simulink model "sim_A3_nonlinear"  (R2022b)
settings: Solver=ode45  StartTime=0.0  StopTime=Tf  RelTol=1e-3
values from neighbouring files (symbols this model uses):
  B = diag([1 2])    [main_A3_nonlinear.m]
  controller = 4    [main_A3_nonlinear.m]
  Cs = [0.4, 0.001 ... (first row only)    [main_A3_nonlinear.m]
  gamma = 1    [main_A3_nonlinear.m]
  K1 = place(A,B,poles_cont)    [main_A3_nonlinear.m]
  K2 = [alpha 0 ... (first row only)    [main_A3_nonlinear.m]
  Ts = 1/1000    (= 0.001)    [main_A3_nonlinear.m]
  x1_o = ro * cos(k * pi/6)    [main_A3_nonlinear.m]
  x2_o = ro * sin(k * pi/6)    [main_A3_nonlinear.m]
undefined symbols (not defined in the file or in its folder): K3
settings Model: Creator=ricardoaguilera  LastModifiedBy=lucien
settings SolverCC: AlgebraicLoopSolver=TrustRegion
settings DataIOCC: ReturnWorkspaceOutputs=off
settings OptimizationCC: LifeSpan=inf
settings DebuggingCC: UnconnectedInputMsg=warning  UnconnectedOutputMsg=warning  UnconnectedLineMsg=warning  SFMachineParentedDataDiag=warning  ArithmeticOperatorsInVariantConditions=warning
settings ModelReferenceCC: EnableRefExpFcnMdlSchedulingChecks=on
settings SFSimCC: CustomCodeUndefinedFunction=UseInterfaceOnly
settings CodeAppCC: StateflowObjectComments=on

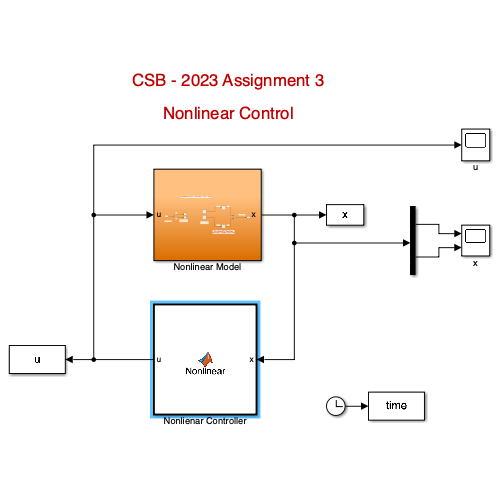
[thumbnail: Simulink's stored preview of the top-level diagram]
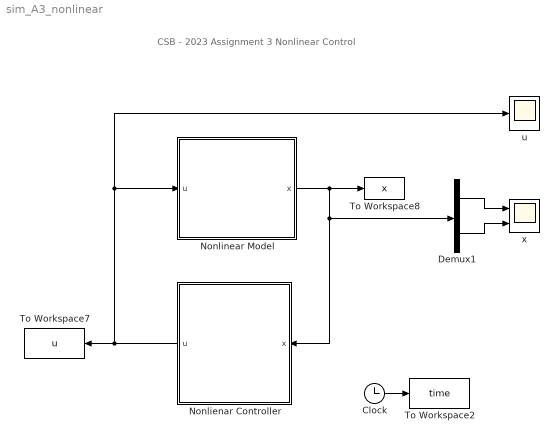
== system sim_A3_nonlinear ==
  note: CSB - 2023 Assignment 3
      |
      | Nonlinear Control
  Clock : Clock
  Demux1 : Demux  Outputs=2
  Nonlienar Controller : MATLAB Function  TreatAsAtomicUnit=on  SystemSampleTime=Ts
  Nonlinear Model : Subsystem
  To Workspace2 : ToWorkspace  VariableName=time  SampleTime=Ts/20
  To Workspace7 : ToWorkspace  VariableName=u  SampleTime=Ts/20
  To Workspace8 : ToWorkspace  VariableName=x  SampleTime=Ts/20
  u : Scope
  x : Scope  NumInputPorts=2
  wires:
  Clock/1 -> To Workspace2/1
  Demux1/2 -> x/2
  Demux1/1 -> x/1
  Nonlienar Controller/1(u) -> Nonlinear Model/1(u), u/1, To Workspace7/1
  Nonlinear Model/1("x ") -> Demux1/1, Nonlienar Controller/1(x), To Workspace8/1

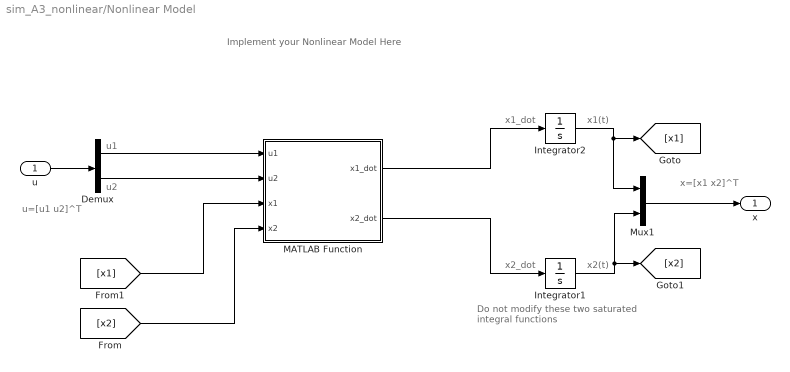
== system sim_A3_nonlinear/Nonlinear Model ==
  note: x=[x1 x2]^T
  note: x1_dot
  note: x2(t)
  note: x1(t)
  note: x2_dot
  note: u=[u1 u2]^T
  note: Implement your Nonlinear Model Here
  note: Do not modify these two
      | saturated integral functions
  note: u1
  note: u2
  u : Inport
  Demux : Demux  Outputs=2
  Integrator1 : Integrator  InitialCondition=x2_o  LimitOutput=on  UpperSaturationLimit=100  LowerSaturationLimit=-100
  Integrator2 : Integrator  InitialCondition=x1_o  LimitOutput=on  UpperSaturationLimit=100  LowerSaturationLimit=-100
  MATLAB Function : MATLAB Function  TreatAsAtomicUnit=on
  Mux1 : Mux  Inputs=2
  "x " : Outport
  wires:
  Integrator1/1 -> [x2], Mux1/2
  Integrator2/1 -> [x1], Mux1/1
  Mux1/1 -> "x "/1
  u/1 -> Demux/1
  MATLAB Function/1(x1_dot) -> Integrator2/1
  MATLAB Function/2(x2_dot) -> Integrator1/1
  Demux/2 -> MATLAB Function/2(u2)
  Demux/1 -> MATLAB Function/1(u1)
  [x1] -> MATLAB Function/3(x1)
  [x2] -> MATLAB Function/4(x2)

== matlab function sim_A3_nonlinear/Nonlinear Model/MATLAB Function ==
  data: u1 input; x1_dot output; u2 input; x1 input; x2 input; x2_dot output
function [x1_dot, x2_dot]= dynamics(u1, u2, x1,x2)

x1_dot = x1*(x1^2 +x2^2) + 2*x1*x2^2 + 6*x2 + u1;
x2_dot = x2*(x1^2 +x2^2) - 2*x1^2*x2 -  2*x1 + 2*u2; 

end

== matlab function sim_A3_nonlinear/Nonlienar Controller ==
  data: x input; u output; Cs parameter; B parameter; gamma parameter; K1 parameter; K2 parameter; K3 parameter; controller parameter
function u = Nonlinear(x, Cs,B, gamma,K1, K2, K3, controller)
% Initializations to define arrays size
% Do not delete
x_k = zeros(2,1);
x1 = 0;
x2 = 0;
Sx = zeros(2,1);
u_k=[0 0]';

%% Measurements
x_k=x;
x1 = x_k(1);
x2 = x_k(2);

switch controller
    %% Implement the required controllers in each case section
    %  Modify all of them as required
    case 1
    %% SFC with closed-loop poles p=[-2, -2]
    
    u_k=-K1*x_k;
    
    case 2
    %% SFC with guaranteed region of attraction ||x||^2 < 3^2
    
    u_k=-K2*x_k;
    
    case 3
    %% Feedback Linearization
    
    v_k=-K3*x_k;
    u_k(1)= v_k(1) - x1*(x1^2 + x2^2) - 2*x1*x2^2;
    u_k(2)= (v_k(2) - x2*(x1^2 + x2^2) + 2*x1^2*x2)/2;
    
    case 4
    %% SMC
    Sx = Cs*x_k; %surface
    
    
    f1 = x1*(x1^2 +x2^2) + 2*x1*x2^2 + 6*x2;
    f2 = x2*(x1^2 +x2^2) - 2*x1^2*x2 -  2*x1;
    f = [f1 f2]';
    
    ueq_k = -(Cs*B)\Cs*f;
    usw_k = -gamma*(Cs*B)\tanh(100*Sx);
    
    u_k = ueq_k + usw_k;

   
end

u = u_k;
